simulink model "Simulation_RAFAEL"  (R2024a)
settings: Solver=ode4  StartTime=0.0  StopTime=10.0  FixedStep=0.001  RelTol=1e-3
InitFcn:
  | init_file
values from neighbouring files (symbols this model uses):
  init_followingDistance = 93.9    [init_file.m]
  init_MASVelocity = 31.3    [init_file.m]
  sampleTime = 0.001    [init_file.m]
libraries: SignalEditorBlockLib x1, dspsrcs4 x1, fuzblock x1
settings Model: Creator=hbf502  LastModifiedBy=hbf502

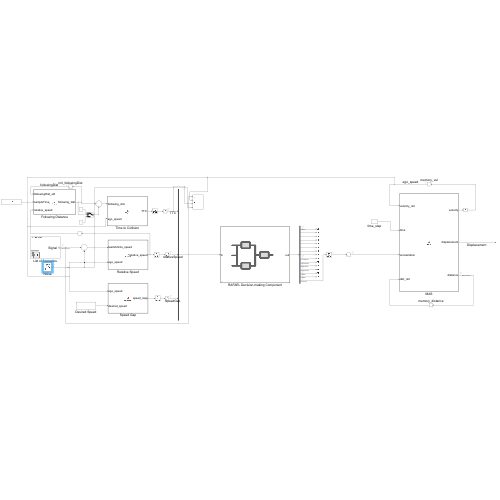
[thumbnail: Simulink's stored preview of the top-level diagram]
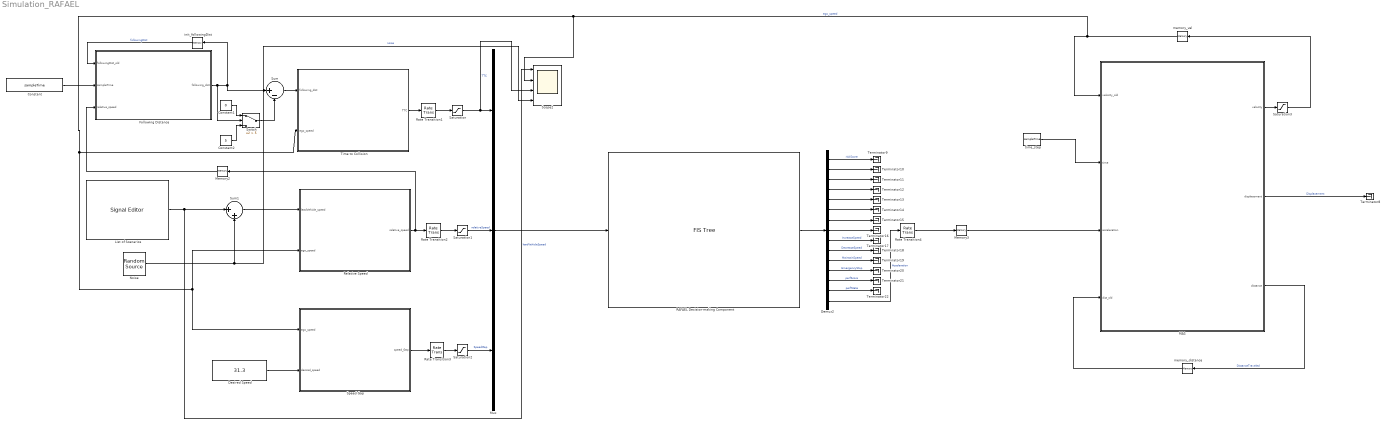
== system Simulation_RAFAEL ==
  Constant : Constant  Value=sampleTime
  Constant1 : Constant  Value=0
  Constant2 : Constant  Value=5
  Demux2 : Demux  Outputs=15
  Desired Speed : Constant  Value=31.3  SampleTime=-1
  Following Distance : MATLAB Function  TreatAsAtomicUnit=on
  List of Scenarios : SignalEditorBlockLib/Signal Editor  FileName=TestScenarios.mat  ActiveScenario=BrakingNAccelerate  ActiveSignal=Signal 1  IsBus=off  OutputBusObjectStr=Bus: BusObject  SampleTime=-1  ZeroCross=off  OutputAfterFinalValue=Setting to zero  Unit=inherit  PreserveSignalName=on  ApplySigPropsToAllScenarios=on  ApplySigPropsToAllSignals=off
  MAS : MATLAB Function  TreatAsAtomicUnit=on
  Memory2 : Memory  InheritSampleTime=on
  Memory3 : Memory  InheritSampleTime=on
  Mux : Mux  Inputs=3
  Noise : dspsrcs4/Random Source  SrcType=Gaussian  MinVal=0  MaxVal=0  MeanVal=0  VarVal=0.1  RepMode=Specify seed  rawSeed=1  IsInherit=off  SampTime=sampleTime  SampFrame=1  OutComplex=Real  DataType=double  SimulateUsing=Interpreted execution
  RAFAEL Decision-making Component : fuzblock/FIS Tree  FIS='fistreeDecisionComponent'  OutputSampleNumber=101  DataType=double  SimulateUsing=Interpreted execution  OutOfRangeInputValueMessage=warning  NoRuleFiredMessage=warning  EmptyOutputFuzzySetMessage=warning
  Rate Transition1 : RateTransition  OutPortSampleTime=monitorUpdateRate
  Rate Transition2 : RateTransition  OutPortSampleTime=monitorUpdateRate
  Rate Transition3 : RateTransition  OutPortSampleTime=monitorUpdateRate
  Rate Transition4 : RateTransition  OutPortSampleTime=sampleTime
  Relative Speed : MATLAB Function  TreatAsAtomicUnit=on
  Saturation : Saturate  UpperLimit=4  LowerLimit=0
  Saturation1 : Saturate  UpperLimit=31.3  LowerLimit=-31.3
  Saturation2 : Saturate  UpperLimit=1  LowerLimit=-1
  Saturation3 : Saturate  UpperLimit=35  LowerLimit=0
  Scope2 : Scope  NumInputPorts=4
  Speed Gap : MATLAB Function  TreatAsAtomicUnit=on
  Sum : Sum  Inputs=|+-
  Sum1 : Sum  Inputs=|++
  Switch : Switch  Criteria=u2 > Threshold  Threshold=5  SaturateOnIntegerOverflow=off  InputSameDT=off
  Terminator{8..22} (15 alike) : Terminator
  Time to Collision : MATLAB Function  TreatAsAtomicUnit=on
  init_followingDist : Memory  InitialCondition=init_followingDistance  InheritSampleTime=on
  memory_distance : Memory  InheritSampleTime=on
  memory_vel : Memory  InitialCondition=init_MASVelocity  InheritSampleTime=on
  time_step : Constant  Value=sampleTime
  wires:
  time_step/1 -> MAS/2(time)
  MAS/1(velocity) -> Saturation3/1
  memory_vel/1 -> Scope2/2, Speed Gap/1(ego_speed), Relative Speed/2(ego_speed), Time to Collision/2(ego_speed), MAS/1(velocity_old)  "ego_speed"
  MAS/3(distance) -> memory_distance/1  "DistanceTraveled"
  memory_distance/1 -> MAS/4(dist_old)
  Time to Collision/1(TTC) -> Rate Transition1/1
  Relative Speed/1(relative_speed) -> Memory2/1, Rate Transition2/1
  Speed Gap/1(speed_Gap) -> Rate Transition3/1
  Desired Speed/1 -> Speed Gap/2(desired_speed)
  Saturation/1 -> Scope2/3, Mux/1  "TTC"
  Saturation1/1 -> Mux/2  "relativeSpeed"
  Saturation2/1 -> Mux/3  "SpeedGap"
  MAS/2(displacement) -> Terminator8/1  "Displacement"
  Following Distance/1(following_dist) -> Switch/2, Sum/1, init_followingDist/1
  init_followingDist/1 -> Following Distance/1(followingDist_old)  "followingDist"
  Constant/1 -> Following Distance/2(sampleTime)
  Saturation3/1 -> memory_vel/1
  Mux/1 -> RAFAEL Decision-making Component/1
  Rate Transition1/1 -> Saturation/1
  Rate Transition2/1 -> Saturation1/1
  Rate Transition3/1 -> Saturation2/1
  Memory2/1 -> Following Distance/3(relative_speed)
  Sum/1 -> Time to Collision/1(following_dist)
  Rate Transition4/1 -> Memory3/1
  RAFAEL Decision-making Component/1 -> Demux2/1
  Demux2/1 -> Terminator9/1  "riskScore"
  Demux2/2 -> Terminator10/1
  Demux2/3 -> Terminator11/1
  Demux2/4 -> Terminator12/1
  Demux2/5 -> Terminator13/1
  Demux2/6 -> Terminator14/1
  Demux2/7 -> Terminator15/1
  Demux2/8 -> Terminator16/1
  Demux2/9 -> Terminator17/1  "IncreaseSpeed"
  Demux2/10 -> Terminator18/1  "DecreaseSpeed"
  Demux2/11 -> Terminator19/1  "MaintainSpeed"
  Demux2/12 -> Terminator20/1  "EmergencyStop"
  Demux2/13 -> Terminator21/1  "perfScore"
  Demux2/14 -> Terminator22/1  "perfState"
  Demux2/15 -> Rate Transition4/1  "Acceleration"
  List of Scenarios/1 -> Scope2/1, Sum1/1  "leadVehicleSpeed"
  Sum1/1 -> Relative Speed/1(leadVehicle_speed)
  Noise/1 -> Sum1/2, Scope2/4  "noise"
  Constant2/1 -> Switch/3
  Constant1/1 -> Switch/1
  Switch/1 -> Sum/2
  Memory3/1 -> MAS/3(acceleration)

== matlab function Simulation_RAFAEL/Time to Collision ==
  data: following_dist input; ego_speed input; TTC output

function TTC  = TTC_calc(following_dist, ego_speed)
    timeToCollision = following_dist/ego_speed;

    TTC = timeToCollision;
end

== matlab function Simulation_RAFAEL/MAS ==
  data: velocity_old input; time input; velocity output; displacement output; acceleration input; distance output; dist_old input

function [velocity,displacement,distance] = vehicle(velocity_old, time, acceleration, dist_old)
    vel = velocity_old + (acceleration * time);
    pos = (velocity_old * time) + (0.5 * acceleration * (time^2));
    dist = dist_old + pos;

    velocity = vel; distance = dist; displacement = pos;
end

== matlab function Simulation_RAFAEL/Relative Speed ==
  data: leadVehicle_speed input; ego_speed input; relative_speed output
function relative_speed  = rel_speed(leadVehicle_speed, ego_speed)
    relSpeed = leadVehicle_speed - ego_speed;
    relative_speed = relSpeed;
end

== matlab function Simulation_RAFAEL/Speed Gap ==
  data: ego_speed input; desired_speed input; speed_Gap output
function speed_Gap  = speedGapCalc(ego_speed, desired_speed)
    speedGap = (ego_speed - desired_speed)/desired_speed;
    speed_Gap = speedGap;
end

== matlab function Simulation_RAFAEL/Following Distance ==
  data: followingDist_old input; sampleTime input; following_dist output; relative_speed input
function following_dist = updateStoppingDistance(followingDist_old, sampleTime, relative_speed)

    dt = sampleTime;
    stopDist = followingDist_old + (relative_speed*dt);
    

    following_dist = stopDist;

    if following_dist < 0
        following_dist = 0;
    end
end
